simulink library "F_Line_block"  (R2015b)
settings: Solver=VariableStepAuto  StartTime=0.0  StopTime=10.0  RelTol=1e-3
settings Model: Creator=altari  LastModifiedBy=altari

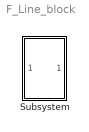
== system F_Line_block ==
  Subsystem : Subsystem

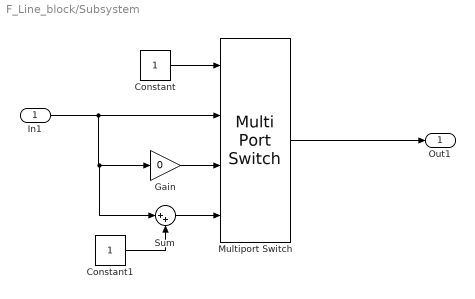
== system F_Line_block/Subsystem ==
  In1 : Inport
  Constant : Constant
  Constant1 : Constant
  Gain : Gain  Gain=0
  Multiport Switch : MultiPortSwitch
  Sum : Sum  Inputs=|++
  Out1 : Outport
  wires:
  Gain/1 -> Multiport Switch/3
  Constant/1 -> Multiport Switch/1
  Constant1/1 -> Sum/2
  Sum/1 -> Multiport Switch/4
  In1/1 -> Sum/1, Gain/1, Multiport Switch/2
  Multiport Switch/1 -> Out1/1
